simulink model "pr742_QPSK_synch_demod"  (R2018b)
settings: Solver=VariableStepAuto  StartTime=0.0  StopTime=50000/fs  RelTol=1e-3
PreLoadFcn:
  | pr741_QPSK_synch_setup;
values from neighbouring files (symbols this model uses):
  fc = 600e3    (= 600000)    [pr741_QPSK_synch_setup.m]
  fe = 400    [pr741_QPSK_synch_setup.m]
  fs = 2.4e6    (= 2400000)    [pr741_QPSK_synch_setup.m]
  interp = fs/Rsyml    (= 48)    [pr741_QPSK_synch_setup.m]
  K1 = (4*d*Bn*T)/(Ko*Kp*(d+1/(4*d)))    (= 0.0444399694694)    [pr741_QPSK_synch_setup.m]
  K2 = (4*(Bn*T)^2)/(Ko*Kp*(d+1/4*d)^2)    (= 7.11325931542e-05)    [pr741_QPSK_synch_setup.m]
  Ko = 0.1    [pr741_QPSK_synch_setup.m]
  Rbit = 100e3    (= 100000)    [pr741_QPSK_synch_setup.m]
libraries: commfilt2 x4, commsynccomp2 x2, commrandsrc3 x1, commdigbbndpm3 x1, dspsigops x1
settings Model: Creator=Григорий Фокин  LastModifiedBy=Григорий Фокин
settings DataIOCC: SaveFormat=Array  SaveOutput=off  SignalLogging=off  SaveTime=off
settings DebuggingCC: AlgebraicLoopMsg=error
settings HardwareCC: ProdBitPerPointer=32  ProdBitPerSizeT=32  ProdBitPerPtrDiffT=32  ProdLargestAtomicFloat=None  ProdIntDivRoundTo=Undefined  ProdEndianess=Unspecified  ProdWordSize=32  ProdHWDeviceType=ASIC/FPGA->ASIC/FPGA  TargetBitPerPointer=64  TargetBitPerSizeT=64  TargetBitPerPtrDiffT=64  TargetLongLongMode=on  TargetIntDivRoundTo=Zero  TargetEndianess=LittleEndian  TargetWordSize=64  TargetHWDeviceType=Custom Processor->MATLAB Host Computer  ProdEqTarget=off

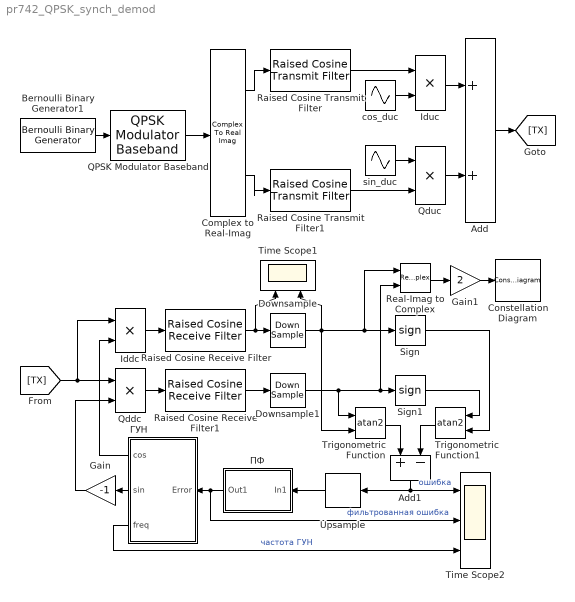
== system pr742_QPSK_synch_demod ==
  Add : Sum
  Add1 : Sum  Inputs=+-
  Bernoulli Binary Generator1 : commrandsrc3/Bernoulli Binary Generator  ProbabilityOfZero=0.5  SeedSource=Auto  Seed=0  SampleTime=1/Rbit  SamplesPerFrame=2  OutputDataType=double  SimulateUsing=Interpreted execution
  Complex to Real-Imag : ComplexToRealImag
  Constellation Diagram : ConstellationDiagram
  Downsample : DownSample  N=interp  RateOptions=Allow multirate processing
  Downsample1 : DownSample  N=interp  RateOptions=Allow multirate processing
  Gain : Gain  Gain=-1
  Gain1 : Gain  Gain=2
  Iddc : Product
  Iduc : Product
  QPSK Modulator Baseband : commdigbbndpm3/QPSK Modulator Baseband  InType=Bit  Enc=Gray  Ph=pi/4  outDtype=Fixed-point  outWordLen=16  outUDDataType=sfix(16)  outFracLenMode=Best precision  outFracLen=15  outDataTypeStr=fixdt(1,16)  outLastDataTypeStr=fixdt(1,16)
  Qddc : Product
  Qduc : Product
  Raised Cosine Receive Filter : commfilt2/Raised Cosine Receive Filter  filtType=Square root  R=0.25  filtSpan=8  N=interp  downFactor=1  downOffset=0  filterGain=1  RateOptions=Allow multirate processing  framing=Mute  checkCoeff=off  variableName=rcRxFilt  currentFiltSpan=8  D=(8)/2  inputOffset=0  sampMode=Mute  saveAsFlag=0  rateMode=Downsampling  checkGain=Normalized  launchFVT=on  roundingMode=Floor  overflowMode=off  coeffDataTypeStr=Inherit: Same word length as input  coeffMin=[]  coeffMax=[]  coeffLastDataTypeStr=Inherit: Same word length as input  accumDataTypeStr=Inherit: Same as product output  accumLastDataTypeStr=Inherit: Same as product output  outputDataTypeStr=Inherit: Same as accumulator  outputMin=[]  outputMax=[]  outputLastDataTypeStr=Inherit: Same as accumulator
  Raised Cosine Receive Filter1 : commfilt2/Raised Cosine Receive Filter  filtType=Square root  R=0.25  filtSpan=8  N=interp  downFactor=1  downOffset=0  filterGain=1  RateOptions=Allow multirate processing  framing=Mute  checkCoeff=off  variableName=rcRxFilt1  currentFiltSpan=8  D=(8)/2  inputOffset=0  sampMode=Mute  saveAsFlag=0  rateMode=Downsampling  checkGain=Normalized  launchFVT=on  roundingMode=Floor  overflowMode=off  coeffDataTypeStr=Inherit: Same word length as input  coeffMin=[]  coeffMax=[]  coeffLastDataTypeStr=Inherit: Same word length as input  accumDataTypeStr=Inherit: Same as product output  accumLastDataTypeStr=Inherit: Same as product output  outputDataTypeStr=Inherit: Same as accumulator  outputMin=[]  outputMax=[]  outputLastDataTypeStr=Inherit: Same as accumulator
  Raised Cosine Transmit Filter : commfilt2/Raised Cosine Transmit Filter  filtType=Square root  R=0.25  filtSpan=8  N=interp  filterGain=1  RateOptions=Allow multirate processing  framing=Mute  checkCoeff=off  variableName=rcTxFilt  checkGain=Normalized  sampMode=Mute  saveAsFlag=0  currentFiltSpan=8  D=(8)/2  launchFVT=on  roundingMode=Floor  overflowMode=off  coeffDataTypeStr=Inherit: Same word length as input  coeffMin=[]  coeffMax=[]  coeffLastDataTypeStr=Inherit: Same word length as input  outputDataTypeStr=Inherit: Same as accumulator  outputMin=[]  outputMax=[]  outputLastDataTypeStr=Inherit: Same as accumulator
  Raised Cosine Transmit Filter1 : commfilt2/Raised Cosine Transmit Filter  filtType=Square root  R=0.25  filtSpan=8  N=interp  filterGain=1  RateOptions=Allow multirate processing  framing=Mute  checkCoeff=off  variableName=rcTxFilt1  checkGain=Normalized  sampMode=Mute  saveAsFlag=0  currentFiltSpan=8  D=(8)/2  launchFVT=on  roundingMode=Floor  overflowMode=off  coeffDataTypeStr=Inherit: Same word length as input  coeffMin=[]  coeffMax=[]  coeffLastDataTypeStr=Inherit: Same word length as input  outputDataTypeStr=Inherit: Same as accumulator  outputMin=[]  outputMax=[]  outputLastDataTypeStr=Inherit: Same as accumulator
  Real-Imag to Complex : RealImagToComplex
  Sign : Signum
  Sign1 : Signum
  Time Scope1 : Scope  NumInputPorts=2
  Time Scope2 : Scope  NumInputPorts=3
  Trigonometric Function : Trigonometry  Operator=atan2
  Trigonometric Function1 : Trigonometry  Operator=atan2
  Upsample : dspsigops/Upsample  N=interp  phase=0  RateOptions=Allow multirate processing  ic=0  mode=Unused parameter value
  cos_duc : Sin  Frequency=(fc+fe)*2*pi  Phase=pi/2  SampleTime=1/fs
  sin_duc : Sin  Frequency=(fc+fe)*2*pi  SampleTime=1/fs
  ГУН : Subsystem  mask{fq=fc, sensitivity=Ko*fs}
      mask prompts: fq "Quiescent Frequency (Гц)"; sensitivity "Sensitivity (Гц/В)"
  ПФ : Subsystem
  wires:
  cos_duc/1 -> Iduc/2
  Complex to Real-Imag/1 -> Raised Cosine Transmit Filter/1
  Qduc/1 -> Add/2
  Iduc/1 -> Add/1
  QPSK Modulator Baseband/1 -> Complex to Real-Imag/1
  Complex to Real-Imag/2 -> Raised Cosine Transmit Filter1/1
  Bernoulli Binary Generator1/1 -> QPSK Modulator Baseband/1
  sin_duc/1 -> Qduc/1
  Raised Cosine Transmit Filter/1 -> Iduc/1
  Raised Cosine Transmit Filter1/1 -> Qduc/2
  Add/1 -> [TX]
  Iddc/1 -> Raised Cosine Receive Filter/1
  Qddc/1 -> Raised Cosine Receive Filter1/1
  [TX] -> Iddc/1, Qddc/1
  ГУН/1(cos) -> Iddc/2
  ГУН/3(freq) -> Time Scope2/3  "частота ГУН"
  ГУН/2(sin) -> Gain/1
  Gain/1 -> Qddc/2
  Raised Cosine Receive Filter/1 -> Time Scope1/1, Downsample/1
  Raised Cosine Receive Filter1/1 -> Downsample1/1
  Downsample/1 -> Real-Imag to Complex/1, Sign/1, Time Scope1/2, Trigonometric Function/2
  Downsample1/1 -> Trigonometric Function/1, Real-Imag to Complex/2, Sign1/1
  Sign/1 -> Trigonometric Function1/2
  Sign1/1 -> Trigonometric Function1/1
  Trigonometric Function/1 -> Add1/1
  Trigonometric Function1/1 -> Add1/2
  ПФ/1(Out1) -> Time Scope2/2, ГУН/1(Error)  "фильтрованная ошибка"
  Upsample/1 -> ПФ/1(In1)
  Add1/1 -> Time Scope2/1, Upsample/1  "ошибка"
  Real-Imag to Complex/1 -> Gain1/1
  Gain1/1 -> Constellation Diagram/1

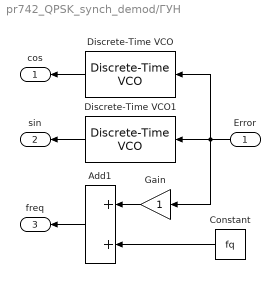
== system pr742_QPSK_synch_demod/ГУН ==
  Error : Inport
  Add1 : Sum
  Constant : Constant  Value=fq
  Discrete-Time VCO : commsynccomp2/Discrete-Time VCO  Ac=1  Fc=fq  Kc=sensitivity  Ph=pi/2  ts=1/fs
      settings: SourceProductName=Communications System Toolbox  SourceProductBaseCode=CM
  Discrete-Time VCO1 : commsynccomp2/Discrete-Time VCO  Ac=1  Fc=fq  Kc=sensitivity  Ph=0  ts=1/fs
      settings: SourceProductName=Communications System Toolbox  SourceProductBaseCode=CM
  Gain : Gain
  cos : Outport
  sin : Outport  Port=2
  freq : Outport  Port=3
  wires:
  Add1/1 -> freq/1
  Discrete-Time VCO/1 -> cos/1
  Error/1 -> Discrete-Time VCO/1, Gain/1, Discrete-Time VCO1/1
  Gain/1 -> Add1/1
  Discrete-Time VCO1/1 -> sin/1
  Constant/1 -> Add1/2

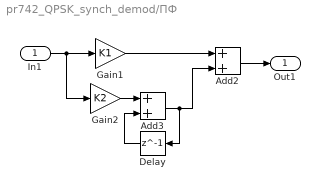
== system pr742_QPSK_synch_demod/ПФ ==
  In1 : Inport
  Add2 : Sum
  Add3 : Sum
  Delay : Delay  DelayLength=1  InitialCondition=0
  Gain1 : Gain  Gain=K1
  Gain2 : Gain  Gain=K2
  Out1 : Outport
  wires:
  Delay/1 -> Add3/2
  Add2/1 -> Out1/1
  Gain2/1 -> Add3/1
  In1/1 -> Gain2/1, Gain1/1
  Add3/1 -> Delay/1, Add2/2
  Gain1/1 -> Add2/1
